simulink model "Model_1_Braking"  (R2019b)
settings: Solver=ode15s  StartTime=0.0  StopTime=inf  MaxStep=0.005  RelTol=1e-3
model workspace (MATLAB code in the model file):
  | ms = 135;
  | mf = 5;
  | mr = 10;
  | m = ms + (mf + mr);
  | a = 0.7;
  | b = 0.7;
  | Cd = 0.8;
  | Af = 1;
  | h_cg = 0.5;
  | kf = 10000;
  | kr = 15000;
  | cf = 5000;
  | cr = 5000;
  | I = 500;
  | kt = 175000;
values from neighbouring files (symbols this model uses):
  brakef = brake_front(i,j)    [Model_1_Braking_Distance.m]
  braker = brake_rear(i,j)    [Model_1_Braking_Distance.m]
libraries: autolibshared x2
(part 1 of 3)
settings Model: Creator=Barath Krishna S  LastModifiedBy=Barath Krishna S

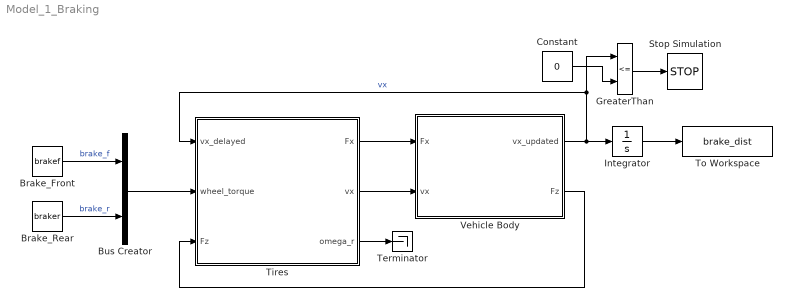
== system Model_1_Braking ==
  Brake_Front : Constant  Value=brakef
  Brake_Rear : Constant  Value=braker
  Bus Creator : BusCreator  Inputs=2
  Constant : Constant  Value=0
  GreaterThan : RelationalOperator  Operator=<=  OutDataTypeStr=boolean  ZeroCross=off  RndMeth=Simplest
  Integrator : Integrator
  Stop Simulation : Stop
  Terminator : Terminator
  Tires : Subsystem
  To Workspace : ToWorkspace  VariableName=brake_dist  SampleTime=-1
      settings: MaxDataPoints=1
  Vehicle Body : Subsystem
  wires:
  Vehicle Body/2(Fz) -> Tires/3(Fz)
  Tires/2(vx) -> Vehicle Body/2(vx)
  Tires/1(Fx) -> Vehicle Body/1(Fx)
  Vehicle Body/1(vx_updated) -> Integrator/1, GreaterThan/1, Tires/1(vx_delayed)  "vx"
  Bus Creator/1 -> Tires/2(wheel_torque)
  Tires/3(omega_r) -> Terminator/1
  Brake_Front/1 -> Bus Creator/1  "brake_f"
  Brake_Rear/1 -> Bus Creator/2  "brake_r"
  Constant/1 -> GreaterThan/2
  GreaterThan/1 -> Stop Simulation/1
  Integrator/1 -> To Workspace/1
